simulink model "Mass_Digital_Obs"  (R2016b)
settings: Solver=ode45  StartTime=0.0  StopTime=100  RelTol=1e-3  EnableMultiTasking=on
InitFcn:
  | param
undefined symbols (not defined in the file or in its folder): drawMassSys, mass_ctrl_obs, P
settings Model: Creator=beard  LastModifiedBy=Jacob
settings DataIOCC: LimitDataPoints=on  SaveFormat=Array  SignalLoggingSaveFormat=ModelDataLogs
settings OptimizationCC: ExpressionDepthLimit=2147483647  InitFltsAndDblsToZero=on  LifeSpan=inf
settings DebuggingCC: UnderspecifiedInitializationDetection=Classic  MergeDetectMultiDrivingBlocksExec=none  SolverPrmCheckMsg=warning  FcnCallInpInsideContextMsg=warning  StateNameClashWarn=warning  SFUnexpectedBacktrackingDiag=warning  SFNoUnconditionalDefaultTransitionDiag=warning  SFExecutionAtInitializationDiag=none
settings HardwareCC: ProdBitPerPointer=32  ProdBitPerSizeT=32  ProdBitPerPtrDiffT=32  ProdLargestAtomicFloat=None  ProdIntDivRoundTo=Undefined  ProdEndianess=Unspecified  ProdWordSize=32  ProdHWDeviceType=32-bit Generic
settings ModelReferenceCC: PropagateSignalLabelsOutOfModel=off
settings GRTTargetCC: TargetLangStandard=C89/C90 (ANSI)  GeneratePreprocessorConditionals=Disable all  CombineOutputUpdateFcns=off  GRTInterface=on
settings ConfigComp: CovMetricSettings=dw  CovHtmlReporting=on  CovSaveCumulativeToWorkspaceVar=on  CovSaveSingleToWorkspaceVar=on  CovExternalEMLEnable=off

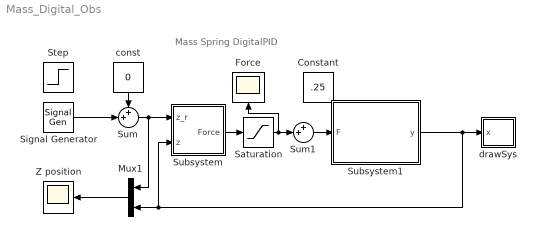
== system Mass_Digital_Obs ==
  note: Mass Spring DigitalPID
  Constant : Constant  Value=.25
  Force : Scope
  Mux1 : Mux  Inputs=2
  Saturation : Saturate  UpperLimit=2  LowerLimit=-2
  Signal Generator : SignalGenerator  WaveForm=square  Amplitude=.5  Frequency=.03
  Step : Step  Time=0  After=.5  SampleTime=0
  Subsystem : Subsystem
  Subsystem1 : Subsystem
  Sum : Sum  Inputs=++|
  Sum1 : Sum  Inputs=++|
  Z position : Scope
  const : Constant  Value=0
  drawSys : Subsystem
  wires:
  Saturation/1 -> Sum1/2, Force/1
  Mux1/1 -> Z position/1
  Subsystem/1(Force) -> Saturation/1
  Sum/1 -> Mux1/1, Subsystem/1(z_r)
  const/1 -> Sum/1
  Subsystem1/1(y) -> Subsystem/2(z), Mux1/2, drawSys/1(x)
  Sum1/1 -> Subsystem1/1(F)
  Signal Generator/1 -> Sum/2

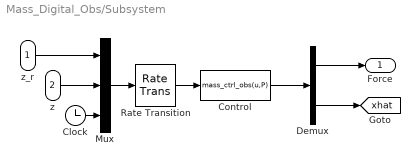
== system Mass_Digital_Obs/Subsystem ==
  z_r : Inport
  z : Inport  Port=2
  Clock : Clock
  Control : MATLABFcn  MATLABFcn=mass_ctrl_obs(u,P)  OutputDimensions=1+2
  Demux : Demux  Outputs=[1;2]
  Mux : Mux  Inputs=3
  Rate Transition : RateTransition  OutPortSampleTime=P.Ts
  Force : Outport
  tag scope: xhat=global
  wires:
  z_r/1 -> Mux/1
  z/1 -> Mux/2
  Mux/1 -> Rate Transition/1
  Rate Transition/1 -> Control/1
  Clock/1 -> Mux/3
  Control/1 -> Demux/1
  Demux/1 -> Force/1
  Demux/2 -> [xhat]

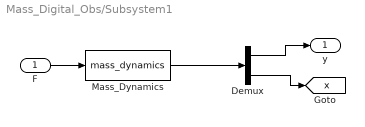
== system Mass_Digital_Obs/Subsystem1 ==
  F : Inport
  Demux : Demux  Outputs=[1;2]
  Mass_Dynamics : S-Function  FunctionName=mass_dynamics  Parameters=P  SFunctionDeploymentMode=off  EnableBusSupport=off
  y : Outport
  tag scope: x=global
  wires:
  F/1 -> Mass_Dynamics/1
  Mass_Dynamics/1 -> Demux/1
  Demux/1 -> y/1
  Demux/2 -> [x]

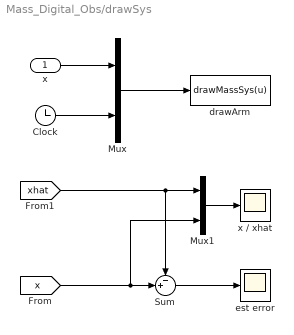
== system Mass_Digital_Obs/drawSys ==
  x : Inport
  Clock : Clock
  Mux : Mux  Inputs=2
  Mux1 : Mux  Inputs=2
  Sum : Sum  Inputs=-+|
  drawArm : MATLABFcn  MATLABFcn=drawMassSys(u)  OutputDimensions=0  SampleTime=0.1
  est error : Scope
  x / xhat : Scope
  wires:
  Mux/1 -> drawArm/1
  x/1 -> Mux/1
  Clock/1 -> Mux/2
  Mux1/1 -> x / xhat/1
  Sum/1 -> est error/1
  [xhat] -> Mux1/1, Sum/1
  [x] -> Mux1/2, Sum/2
